simulink model "doc_carrier"  (R2014a)
settings: Solver=ode45  StartTime=0.0  StopTime=inf  RelTol=1e-3
undefined symbols (not defined in the file or in its folder): commblksprivate, gcbh, Info, rcfiltgaincompat
libraries: commdigbbndpm3 x2, commfilt2 x2, commchan3 x1, commsink2 x1, commphrec2 x1, commrflib2 x1, commrandsrc2 x1, commtimrec2 x1, dspsigops x1
settings Model: Creator=The MathWorks Inc.
settings DataIOCC: SignalLoggingSaveFormat=ModelDataLogs  SaveOutput=off  SaveTime=off  SignalLoggingName=logsOut
settings OptimizationCC: ExpressionDepthLimit=2147483647  InitFltsAndDblsToZero=on
settings DebuggingCC: SaveWithParameterizedLinksMsg=none  UnderspecifiedInitializationDetection=Classic  CheckExecutionContextPreStartOutputMsg=on  CheckExecutionContextRuntimeOutputMsg=on  SignalResolutionControl=TryResolveAllWithWarning  SolverPrmCheckMsg=none  InheritedTsInSrcMsg=none  MultiTaskDSMMsg=warning  MultiTaskCondExecSysMsg=none  SigSpecEnsureSampleTimeMsg=none  FcnCallInpInsideContextMsg=UseLocalSettings  StateNameClashWarn=warning  StrictBusMsg=None
settings HardwareCC: ProdHWDeviceType=Specified
settings ModelReferenceCC: UpdateModelReferenceTargets=IfOutOfDate
settings RTWCC: IncludeERTFirstTime=on
settings CodeAppCC: MangleLength=5
settings GRTTargetCC: TargetFcnLib=ansi_tfl_tmw.mat  CombineOutputUpdateFcns=off  GRTInterface=on

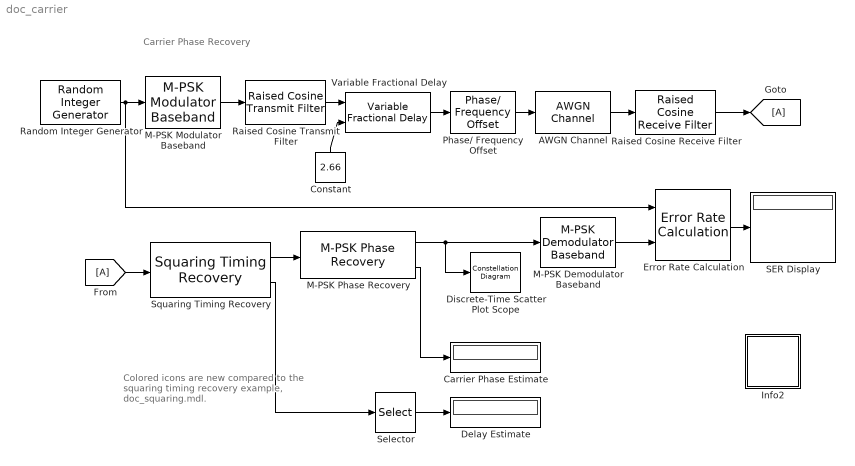
== system doc_carrier ==
  note: Carrier Phase Recovery
  note: Colored icons are new compared
      | to the squaring timing recovery
      | example, doc_squaring.mdl.
  AWGN Channel : commchan3/AWGN Channel  InputProcessing=Columns as channels (frame based)  seed=67  noiseMode="Signal to noise ratio  (SNR)"  EbNodB=10  EsNodB=10  SNRdB=40  bitsPerSym=1  Ps=1  Tsym=1  variance=1
  Carrier Phase Estimate : Display
  Constant : Constant  Value=2.66
  Delay Estimate : Display
  Discrete-Time Scatter Plot Scope : ConstellationDiagram  Tag=ScatterPlot
  Error Rate Calculation : commsink2/Error Rate Calculation  N=2*4  st_delay=500  cp_mode=Entire frame  subframe=[]  PMode=Port  WsName=ErrorVec  RsMode2=off  stop=off  numErr=100  maxBits=1e6
  Info2 : Subsystem  AncestorBlock=commblksprivate/Info  mask(Info){}
      settings: OpenFcn=helpview([docroot '/toolbox/comm/comm.map'], 'doc_carrier')
      mask Display: disp('Info')
  M-PSK Demodulator Baseband : commdigbbndpm3/M-PSK Demodulator Baseband  M=16  Ph=0  Dec=Binary  Mapping=[0:7]  OutType=Integer  DecType=Hard decision  VarSource=Dialog  Variance=1  outDtype1=double  outDtype2=double  derotateFactorWordLen=16
  M-PSK Modulator Baseband : commdigbbndpm3/M-PSK Modulator Baseband  M=16  InType=Integer  Enc=Binary  Mapping=[0:7]  Ph=0  outDtype=double  outWordLen=16  outUDDataType=sfix(16)  outFracLenMode=Best precision  outFracLen=15
  M-PSK Phase Recovery : commphrec2/M-PSK Phase Recovery  M=16  intPeriod=500
  Phase/ Frequency Offset : commrflib2/Phase// Frequency Offset  phaseOffset=10  freqPort=off  freqOffset=0
  Raised Cosine Receive Filter : commfilt2/Raised Cosine Receive Filter  filtType=Square root  N=8  filtSpan=2*(4)  currentFiltSpan=2*(4)  D=4  R=0.2  sampMode=Mute  saveAsFlag=0  rateMode=Downsampling  downFactor=1  downOffset=0  framing=Maintain input frame rate  InputProcessing=Columns as channels (frame based)  checkGain=Normalized  filterGain=rcfiltgaincompat(gcbh)  checkCoeff=off  variableName=rcRxFilt  launchFVT=off  roundingMode=Floor  overflowMode=off
  Raised Cosine Transmit Filter : commfilt2/Raised Cosine Transmit Filter  filtType=Square root  filtSpan=2*(4)  currentFiltSpan=2*(4)  D=4  R=0.2  sampMode=Mute  saveAsFlag=0  N=8  framing=Maintain input frame rate  InputProcessing=Columns as channels (frame based)  checkGain=Normalized  filterGain=rcfiltgaincompat(gcbh)  checkCoeff=off  variableName=rcTxFilt  launchFVT=off  roundingMode=Floor  overflowMode=off
  Random Integer Generator : commrandsrc2/Random Integer Generator  mul=16  seed=37  Ts=1/100  frameBased=on  sampPerFrame=100  orient=off  outDataType=double
  SER Display : Display
  Selector : Selector  InputPortWidth=100
  Squaring Timing Recovery : commtimrec2/Squaring Timing Recovery  numSymb=100  sampPerSymb=8
  Variable Fractional Delay : dspsigops/Variable Fractional Delay  mode=OBSOLETE  modeActive=Linear  dmax=100  InputProcessing=Columns as channels (frame based)  L=4  FarrowL=4  R=10  alpha=1  ic=0  fallbackFIR=Clip to the minimum value necessary for centered kernel  fallbackFarrow=Clip to the minimum value necessary for centered kernel  noDFT=off  roundingMode=Zero  overflowMode=off
  wires:
  Random Integer Generator/1 -> Error Rate Calculation/1, M-PSK Modulator Baseband/1
  M-PSK Modulator Baseband/1 -> Raised Cosine Transmit Filter/1
  Raised Cosine Receive Filter/1 -> [A]
  AWGN Channel/1 -> Raised Cosine Receive Filter/1
  Constant/1 -> Variable Fractional Delay/2
  Raised Cosine Transmit Filter/1 -> Variable Fractional Delay/1
  Variable Fractional Delay/1 -> Phase/ Frequency Offset/1
  Squaring Timing Recovery/2 -> Selector/1
  Selector/1 -> Delay Estimate/1
  M-PSK Demodulator Baseband/1 -> Error Rate Calculation/2
  Error Rate Calculation/1 -> SER Display/1
  [A] -> Squaring Timing Recovery/1
  Phase/ Frequency Offset/1 -> AWGN Channel/1
  Squaring Timing Recovery/1 -> M-PSK Phase Recovery/1
  M-PSK Phase Recovery/1 -> Discrete-Time Scatter Plot Scope/1, M-PSK Demodulator Baseband/1
  M-PSK Phase Recovery/2 -> Carrier Phase Estimate/1

== system doc_carrier/Info2 ==
